simulink model "ur5_simulink_ros2_pbvs_pid"  (R2023b)
settings: Solver=FixedStepAuto  StartTime=0.0  StopTime=inf  FixedStep=0.04  RelTol=1e-3
model workspace (MAT data in the model file):
  SL_ROS_VariableLengthArrays_MaxSizes.CommonInfo.ArrayTruncateAction = 'EmitWarning'
  SL_ROS_VariableLengthArrays_MaxSizes.MsgTypeMap = containers.Map
  SL_ROS_VariableLengthArrays_MaxSizes.MsgTypeMap.serialization.keys = {'example_interfaces/Float64MultiArray'}
  SL_ROS_VariableLengthArrays_MaxSizes.MsgTypeMap.serialization.values{1}.PropertyName = 'data'
  SL_ROS_VariableLengthArrays_MaxSizes.MsgTypeMap.serialization.values{1}.DataType = 'double'
  SL_ROS_VariableLengthArrays_MaxSizes.MsgTypeMap.serialization.values{1}.MaxLength = 1
  SL_ROS_VariableLengthArrays_MaxSizes.MsgTypeMap.serialization.uniformity = 0
  SL_ROS_VariableLengthArrays_MaxSizes.MsgTypeMap.serialization.keyType = 'char'
  SL_ROS_VariableLengthArrays_MaxSizes.MsgTypeMap.serialization.valueType = 'any'
undefined symbols (not defined in the file or in its folder): data, data_SL_Info
libraries: ros2lib x8, robotmaniplib x3, robotcorelib x1
settings Model: SimulationMode=accelerator  Creator=81232  LastModifiedBy=ias-lab-701
settings OptimizationCC: EnhancedBackFolding=on  PassReuseOutputArgsAs=Individual arguments  ZeroExternalMemoryAtStartup=off  ZeroInternalMemoryAtStartup=off  MaxStackSize=64  OptimizeBlockOrder=speed  DifferentSizesBufferReuse=on  OptimizationCustomize=off  EfficientTunableParamExpr=on
settings DebuggingCC: ParameterTunabilityLossMsg=error
settings ModelReferenceCC: EnableRefExpFcnMdlSchedulingChecks=on
settings SFSimCC: MATLABDynamicMemAlloc=off
settings RTWCC: Description=Embedded Coder  SystemTargetFile=ert.tlc  HardwareBoard=Robot Operating System 2 (ROS 2)  TLCOptions="-aInlineSetEventsForThisBaseRateFcn=TLC_FALSE -aSuppressMultiTaskScheduler=TLC_FALSE  -aRateBasedStepFcn=0"  TemplateMakefile=ert_default_tmf  Toolchain=Colcon Tools  TargetLang=C++
settings CodeAppCC: ForceParamTrailComments=on  IgnoreCustomStorageClasses=off  OperatorAnnotations=on  SimulinkDataObjDesc=on  SFDataObjDesc=on  InsertBlockDesc=on
settings ERTTargetCC: CodeInterfacePackaging=C++ class  RootIOFormat=Structure reference

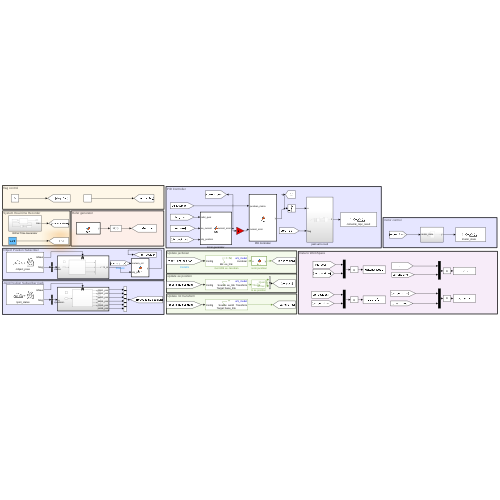
[thumbnail: Simulink's stored preview of the top-level diagram]
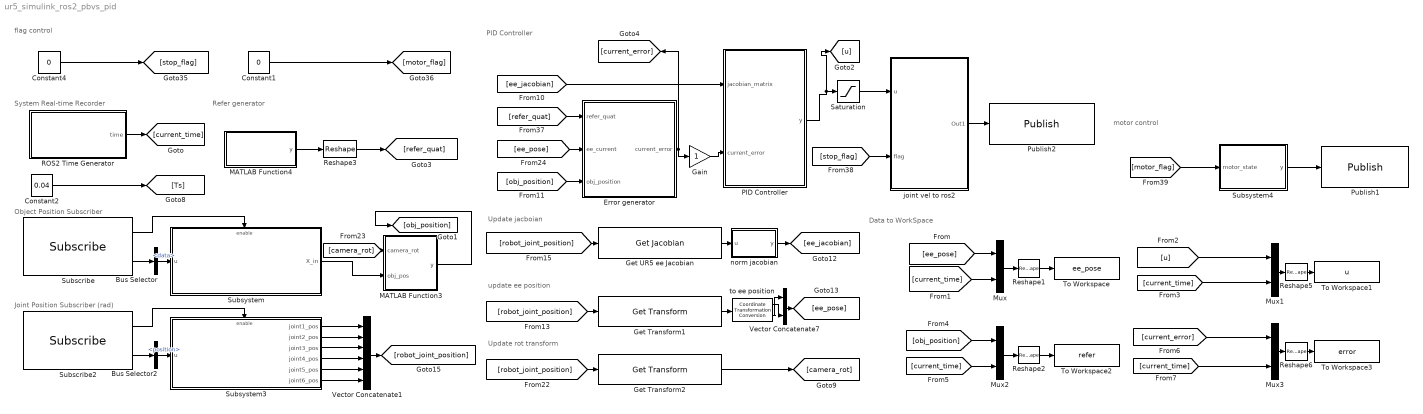
== system ur5_simulink_ros2_pbvs_pid ==
  note: PID Controller
  note: update ee position
  note: Joint Position Subscriber (rad)
  note: Refer generator
  note: Data to WorkSpace
  note: System Real-time Recorder
  note: Object Position Subscriber
  note: Update jacboian
  note: Update rot transform
  note: flag control
  note: motor control
  Bus Selector : BusSelector  OutputSignals=data
  Bus Selector2 : BusSelector  OutputSignals=position
  Constant1 : Constant  Value=0
  Constant2 : Constant  Value=0.04
  Constant4 : Constant  Value=0
  Error generator : MATLAB Function  TreatAsAtomicUnit=on
  Gain : Gain
  Get Transform1 : robotmaniplib/Get Transform  RigidBodyTree=ur5_model  SourceBody=ee_link  TargetBody=base_link  SimulateUsing=Interpreted execution
  Get Transform2 : robotmaniplib/Get Transform  RigidBodyTree=ur5_model  SourceBody=world  TargetBody=base_link  SimulateUsing=Interpreted execution
  Get UR5 ee Jacobian : robotmaniplib/Get Jacobian  RigidBodyTree=ur5_model  EndEffector=ee_link  SimulateUsing=Interpreted execution
  MATLAB Function3 : MATLAB Function  TreatAsAtomicUnit=on
  MATLAB Function4 : MATLAB Function  TreatAsAtomicUnit=on
  Mux{,1..3} (4 alike) : Mux  Inputs=2
  PID Controller : MATLAB Function  TreatAsAtomicUnit=on
  Publish1 : ros2lib/Publish  topicSource=Select from ROS network  topic=/motor_state  messageType=std_msgs/Int64  QOSHistory=Keep last  QOSDepth=1  QOSReliability=Reliable  QOSDurability=Volatile
      settings: LibrarySourceBlock=roslib/ROS 2/Publish
  Publish2 : ros2lib/Publish  topicSource=Select from ROS network  topic=/simulink_mpc_result  messageType=std_msgs/Float64MultiArray  QOSHistory=Keep last  QOSDepth=1  QOSReliability=Reliable  QOSDurability=Volatile
      settings: LibrarySourceBlock=roslib/ROS 2/Publish
  ROS2 Time Generator : Subsystem
  Reshape1 : Reshape  OutputDimensionality=Customize  OutputDimensions=[8]
  Reshape2 : Reshape  OutputDimensionality=Customize  OutputDimensions=[4]
  Reshape3 : Reshape  OutputDimensions=[1,7]
  Reshape5 : Reshape  OutputDimensionality=Customize  OutputDimensions=[7]
  Reshape6 : Reshape  OutputDimensionality=Customize  OutputDimensions=[7]
  Saturation : Saturate  LinearizeAsGain=off
  Subscribe : ros2lib/Subscribe  topicSource=Select from ROS network  topic=/object_pose  messageType=std_msgs/Float64MultiArray  sampleTime=-1  QOSHistory=Keep last  QOSDepth=1  QOSReliability=Reliable  QOSDurability=Volatile
  Subscribe2 : ros2lib/Subscribe  topicSource=Select from ROS network  topic=/joint_states  messageType=sensor_msgs/JointState  sampleTime=-1  QOSHistory=Keep last  QOSDepth=1  QOSReliability=Reliable  QOSDurability=Volatile
  Subsystem : Subsystem
  Subsystem3 : Subsystem
  Subsystem4 : Subsystem
  To Workspace : ToWorkspace  VariableName=ee_pose  SaveFormat=Timeseries  SampleTime=-1
  To Workspace1 : ToWorkspace  VariableName=u  SaveFormat=Timeseries  SampleTime=-1
  To Workspace2 : ToWorkspace  VariableName=refer  SaveFormat=Timeseries  SampleTime=-1
  To Workspace3 : ToWorkspace  VariableName=error  SaveFormat=Timeseries  SampleTime=-1
  Vector Concatenate1 : Concatenate  NumInputs=6
  Vector Concatenate7 : Concatenate
  joint vel to ros2 : Subsystem
  norm jacobian : MATLAB Function  TreatAsAtomicUnit=on
  to ee position : robotcorelib/Coordinate Transformation Conversion  InputRepresentation=Homogeneous Transformation  InputEulerSequence=ZYX  ShowTrVecInputPort=on  OutputRepresentation=Quaternion  OutputEulerSequence=ZYX  ShowTrVecOutputPort=on  SimulateUsing=Interpreted execution
  wires:
  Bus Selector/1 -> Subsystem/1(u)  "<data>"
  Subscribe/2 -> Bus Selector/1
  Subscribe/1 -> Subsystem/Enable
  ROS2 Time Generator/1(time) -> [current_time]
  [ee_pose] -> Mux/1
  [current_time] -> Mux/2
  [current_time] -> Mux1/2
  [current_time] -> Mux2/2
  Mux2/1 -> Reshape2/1
  [current_time] -> Mux3/2
  Mux3/1 -> Reshape6/1
  [current_error] -> Mux3/1
  [u] -> Mux1/1
  Mux1/1 -> Reshape5/1
  Reshape5/1 -> To Workspace1/1
  Reshape6/1 -> To Workspace3/1
  Subscribe2/2 -> Bus Selector2/1
  Bus Selector2/1 -> Subsystem3/1(u)  "<position>"
  Subscribe2/1 -> Subsystem3/Enable
  Subsystem3/1(joint1_pos) -> Vector Concatenate1/1
  Subsystem3/2(joint2_pos) -> Vector Concatenate1/2
  Subsystem3/3(joint3_pos) -> Vector Concatenate1/3
  Subsystem3/4(joint4_pos) -> Vector Concatenate1/4
  Subsystem3/5(joint5_pos) -> Vector Concatenate1/5
  Subsystem3/6(joint6_pos) -> Vector Concatenate1/6
  norm jacobian/1(y) -> [ee_jacobian]
  Get UR5 ee Jacobian/1 -> norm jacobian/1(u)
  [robot_joint_position] -> Get UR5 ee Jacobian/1
  [robot_joint_position] -> Get Transform1/1
  Vector Concatenate1/1 -> [robot_joint_position]
  Mux/1 -> Reshape1/1
  Reshape1/1 -> To Workspace/1
  Reshape2/1 -> To Workspace2/1
  [obj_position] -> Mux2/1
  Constant2/1 -> [Ts]
  Get Transform2/1 -> [camera_rot]
  MATLAB Function3/1(y) -> [obj_position]
  [camera_rot] -> MATLAB Function3/1(camera_rot)
  Subsystem/1(X_in) -> MATLAB Function3/2(obj_pos)
  Reshape3/1 -> [refer_quat]
  MATLAB Function4/1(y) -> Reshape3/1
  [refer_quat] -> Error generator/1(refer_quat)
  Get Transform1/1 -> to ee position/1
  to ee position/1 -> Vector Concatenate7/2
  to ee position/2 -> Vector Concatenate7/1
  Vector Concatenate7/1 -> [ee_pose]
  [ee_jacobian] -> PID Controller/1(jacobian_matrix)
  [obj_position] -> Error generator/3(obj_position)
  [ee_pose] -> Error generator/2(ee_current)
  Saturation/1 -> joint vel to ros2/1(u)
  joint vel to ros2/1(Out1) -> Publish2/1
  PID Controller/1(y) -> Saturation/1, [u]
  Constant4/1 -> [stop_flag]
  [stop_flag] -> joint vel to ros2/2(flag)
  Error generator/1(current_error) -> [current_error], Gain/1
  Gain/1 -> PID Controller/2(current_error)
  Subsystem4/1(y) -> Publish1/1
  [motor_flag] -> Subsystem4/1(motor_state)
  Constant1/1 -> [motor_flag]
  [robot_joint_position] -> Get Transform2/1

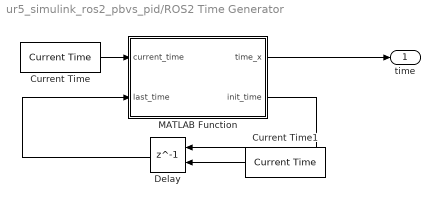
== system ur5_simulink_ros2_pbvs_pid/ROS2 Time Generator ==
  Current Time : ros2lib/Current Time  OutputFormat=double  SampleTime=-1  ModelName=ur5_simulink_ros2_pbvs_pid
      settings: LibrarySourceBlock=roslib/ROS 2/Current Time
  Current Time1 : ros2lib/Current Time  OutputFormat=double  SampleTime=-1  ModelName=ur5_simulink_ros2_pbvs_pid
      settings: LibrarySourceBlock=roslib/ROS 2/Current Time
  Delay : Delay  DelayLength=1  InitialConditionSource=Input port
      settings: InputPortMap=u0,p4
  MATLAB Function : MATLAB Function  TreatAsAtomicUnit=on
  time : Outport
  wires:
  Delay/1 -> MATLAB Function/2(last_time)
  Current Time1/1 -> Delay/2
  MATLAB Function/2(init_time) -> Delay/1
  Current Time/1 -> MATLAB Function/1(current_time)
  MATLAB Function/1(time_x) -> time/1

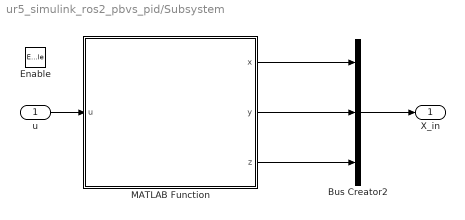
== system ur5_simulink_ros2_pbvs_pid/Subsystem ==
  u : Inport
  Enable : EnablePort
  Bus Creator2 : BusCreator  Inputs=3
  MATLAB Function : MATLAB Function  TreatAsAtomicUnit=on
  X_in : Outport
  wires:
  MATLAB Function/2(y) -> Bus Creator2/2
  MATLAB Function/1(x) -> Bus Creator2/1
  MATLAB Function/3(z) -> Bus Creator2/3
  u/1 -> MATLAB Function/1(u)
  Bus Creator2/1 -> X_in/1

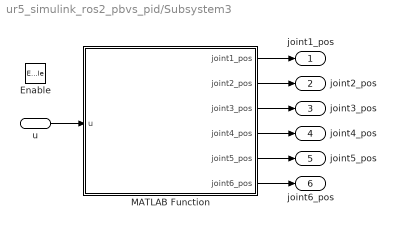
== system ur5_simulink_ros2_pbvs_pid/Subsystem3 ==
  u : Inport
  Enable : EnablePort
  MATLAB Function : MATLAB Function  TreatAsAtomicUnit=on
  joint1_pos : Outport
  joint2_pos : Outport  Port=2
  joint3_pos : Outport  Port=3
  joint4_pos : Outport  Port=4
  joint5_pos : Outport  Port=5
  joint6_pos : Outport  Port=6
  wires:
  u/1 -> MATLAB Function/1(u)
  MATLAB Function/1(joint1_pos) -> joint1_pos/1
  MATLAB Function/2(joint2_pos) -> joint2_pos/1
  MATLAB Function/3(joint3_pos) -> joint3_pos/1
  MATLAB Function/4(joint4_pos) -> joint4_pos/1
  MATLAB Function/5(joint5_pos) -> joint5_pos/1
  MATLAB Function/6(joint6_pos) -> joint6_pos/1

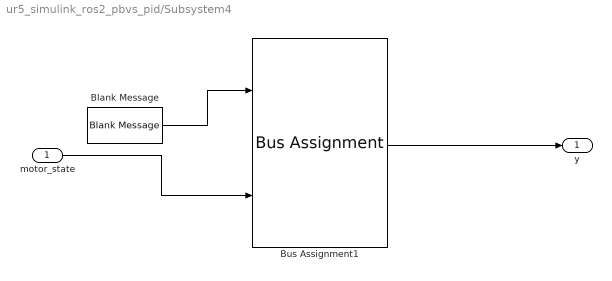
== system ur5_simulink_ros2_pbvs_pid/Subsystem4 ==
  motor_state : Inport
  Blank Message : ros2lib/Blank Message  messageClass=Message  entityType=std_msgs/Int64  messageType=std_msgs/Int64  SampleTime=inf
  Bus Assignment1 : BusAssignment  AssignedSignals=data
  y : Outport
  wires:
  Blank Message/1 -> Bus Assignment1/1
  Bus Assignment1/1 -> y/1
  motor_state/1 -> Bus Assignment1/2

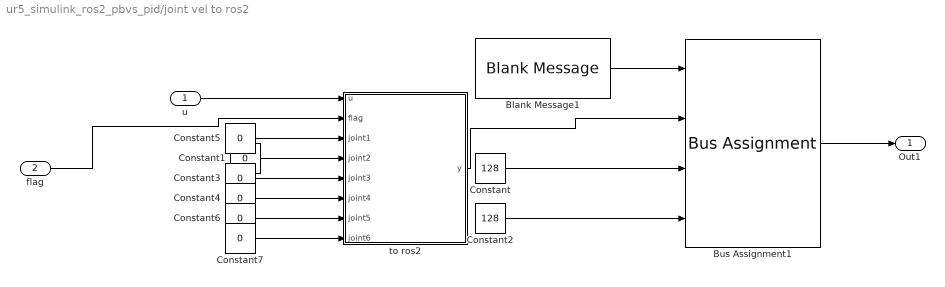
== system ur5_simulink_ros2_pbvs_pid/joint vel to ros2 ==
  u : Inport
  flag : Inport  Port=2
  Blank Message1 : ros2lib/Blank Message  messageClass=Message  entityType=std_msgs/Float64MultiArray  messageType=std_msgs/Float64MultiArray  SampleTime=inf
      settings: LibrarySourceBlock=roslib/ROS 2/Blank Message
  Bus Assignment1 : BusAssignment  AssignedSignals=data,data_SL_Info.CurrentLength,data_SL_Info.ReceivedLength
  Constant : Constant  Value=128  OutDataTypeStr=uint32
  Constant{1,3..7} (6 alike) : Constant  Value=0
  Constant2 : Constant  Value=128  OutDataTypeStr=uint32
  to ros2 : MATLAB Function  TreatAsAtomicUnit=on
  Out1 : Outport
  wires:
  u/1 -> to ros2/1(u)
  Constant2/1 -> Bus Assignment1/4
  Constant/1 -> Bus Assignment1/3
  Blank Message1/1 -> Bus Assignment1/1
  Bus Assignment1/1 -> Out1/1
  Constant5/1 -> to ros2/3(joint1)
  Constant1/1 -> to ros2/4(joint2)
  Constant3/1 -> to ros2/5(joint3)
  Constant4/1 -> to ros2/6(joint4)
  Constant6/1 -> to ros2/7(joint5)
  Constant7/1 -> to ros2/8(joint6)
  flag/1 -> to ros2/2(flag)
  to ros2/1(y) -> Bus Assignment1/2

== matlab function ur5_simulink_ros2_pbvs_pid/Subsystem/MATLAB Function ==
  data: u input; x output; y output; z output
function [x,y,z]= fcn(u)
x = u(1);
y = u(2);
z = u(3);

== matlab function ur5_simulink_ros2_pbvs_pid/ROS2 Time Generator/MATLAB Function ==
  data: current_time input; last_time input; time_x output; init_time output
function [time_x,init_time] = fcn(current_time, last_time)
init_time = last_time;
time_x = current_time-last_time;

== matlab function ur5_simulink_ros2_pbvs_pid/Error generator ==
  data: refer_quat input; ee_current input; obj_position input; current_error output
function current_error  = fcn(refer_quat, ee_current, obj_position)
    position_error = zeros(3,1);
    current_quat = ee_current(4:7);
    ref_quat = refer_quat;
    % sym_ref = [0,-ref_quat(4),ref_quat(3);ref_quat(4),0,-ref_quat(2);-ref_quat(3),ref_quat(2),0];
    % current_error_quat =current_quat(1)*ref_quat(2:4)-ref_quat(1)*current_quat(2:4)-sym_ref*current_quat(2:4);
    w_e = current_quat(1);
    x_e = current_quat(2);
    y_e = current_quat(3);
    z_e = current_quat(4);
    w_d = ref_quat(1);
    x_d = ref_quat(2);
    y_d = ref_quat(3);
    z_d = ref_quat(4);
    current_error_quat = w_e*[x_d;y_d;z_d]-w_d*[x_e;y_e;z_e]-[0,-z_d,y_d;z_d,0,-x_d;-y_d,x_d,0]*[x_e;y_e;z_e];
    position_error(1) = -0.1-1*(ee_current(1)-obj_position(1));
    position_error(2) = -0.02-1*(ee_current(2)-obj_position(2));
    position_error(3) = 0.5-1*(ee_current(3)-obj_position(3));
    current_error = [1*position_error; 0.3*current_error_quat];% x y z

end

== matlab function ur5_simulink_ros2_pbvs_pid/PID Controller ==
  data: jacobian_matrix input; y output; current_error input
function y = fcn(jacobian_matrix, current_error)
    y = jacobian_matrix\current_error;
end

== matlab function ur5_simulink_ros2_pbvs_pid/MATLAB Function3 ==
  data: camera_rot input; obj_pos input; y output
function y = fcn(camera_rot, obj_pos)
    temp_pos = [obj_pos(1);obj_pos(2);obj_pos(3);1];
    new_pos = camera_rot*temp_pos;
    y = new_pos(1:3);
end

== matlab function ur5_simulink_ros2_pbvs_pid/joint vel to ros2/to ros2 ==
  data: u input; flag input; y output; joint1 input; joint2 input; joint3 input; joint4 input; joint5 input; joint6 input
function y  = fcn(u,flag, joint1, joint2, joint3, joint4, joint5, joint6)
    y = zeros(128,1);
    if(flag==0)
        y(1) = u(1);
        y(2) = u(2);
        y(3) = u(3);
        y(4) = u(4);
        y(5) = u(5);
        y(6) = u(6);
    else
        y(1) = joint1;
        y(2) = joint2;
        y(3) = joint3;
        y(4) = joint4;
        y(5) = joint5;
        y(6) = joint6;
    end
end

== matlab function ur5_simulink_ros2_pbvs_pid/norm jacobian ==
  data: u input; y output size=[6,6]
function y = fcn(u)
firstThreeColumns =u(1:3, :);
lastThreeColumns = u(4:6, :);
y = [lastThreeColumns;firstThreeColumns];

== matlab function ur5_simulink_ros2_pbvs_pid/Subsystem3/MATLAB Function ==
  data: u input; joint1_pos output; joint2_pos output; joint3_pos output; joint4_pos output; joint5_pos output; joint6_pos output
function [joint1_pos,joint2_pos,joint3_pos,joint4_pos,joint5_pos,joint6_pos] = fcn(u)
joint1_pos = u(6);
joint2_pos = u(1);
joint3_pos = u(2);
joint4_pos = u(3);
joint5_pos = u(4);
joint6_pos = u(5);

== matlab function ur5_simulink_ros2_pbvs_pid/MATLAB Function4 ==
  data: y output
function y = fcn()
    y =zeros(1,4);
    y(1) =  0.7071;
    y(2) =  0.0001;
    y(3) =  0.7071;
    y(4) =  -0.0000;
end
